simulink model "SingleHip_R2013a"  (R2013a)
settings: Solver=FixedStepDiscrete  StartTime=0.0  StopTime=inf  FixedStep=0.001  MaxStep=0.001  RelTol=1e-3
libraries: xpcethercatlib x21, dspswit3 x1
settings Model: xpc_rtwmakecfg_data=_xpcethercatlib_  BufferReuse=off  Creator=bgbuss  LastModifiedBy=bgbuss
settings OptimizationCC: BlockReduction=off  OptimizeBlockIOStorage=off  BufferReuse=off  ExpressionFolding=off  LocalBlockOutputs=off
settings DebuggingCC: UnderspecifiedInitializationDetection=Simplified
settings HardwareCC: ProdIntDivRoundTo=Zero  ProdEndianess=LittleEndian  ProdHWDeviceType=Generic->32-bit x86 compatible
settings RTWCC: SystemTargetFile=xpctarget.tlc  TemplateMakefile=xpc_default_tmf  Description=xPC Target  ProcessScript=xpctarget_make_rtw_hook  RTWCompilerOptimization=On
settings CodeAppCC: MATLABSourceComments=on
settings xpcTargetCC: TargetFcnLib=ansi_tfl_table_tmw.mat  CodeReplacementLibrary=XPC_BLAS  ParMdlRefBuildCompliant=on  ConcurrentExecutionCompliant=on  CombineSignalStateStructs=off  MATLABClassNameForMDSCustomization=xpcAperiodicCustomization  GRTInterface=on  GenerateAllocFcn=off  RL32LogBufSizeModifier=100000000  xPCTaskExecutionProfile=off  xPCRL32EventNumber=5000  xPCisModelTimeout=off  xPCModelTimeoutSecs=20  xPCLoadParamSetFile=off  xPCConcurrentTasks=off  xPCEnableSFAnimation=off

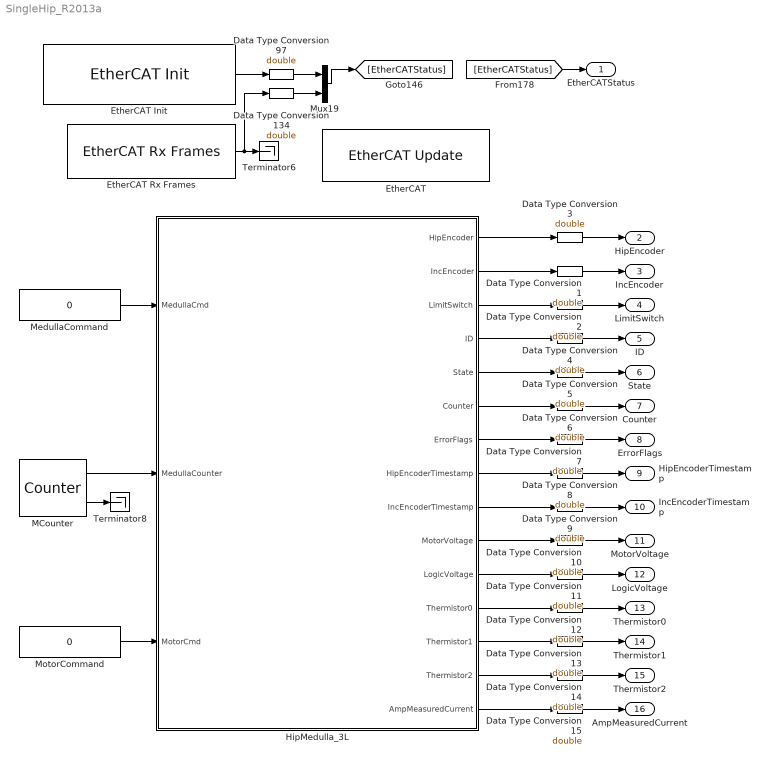
== system SingleHip_R2013a ==
  Data Type Conversion{1..15,97,134} (17 alike) : DataTypeConversion  OutDataTypeStr=double
  EtherCAT : xpcethercatlib/EtherCAT Update   Priority=4  device_id=0  task_id_list=[1]  task_rates=[1]  task_priorities=[1500]
  "EtherCAT Init " : xpcethercatlib/EtherCAT Init   Priority=0  config_file='20140605FullWithMicrostrainDC-eni.xml'  device_id=0  pci_bus=10  pci_slot=0  enaDC=on  errRptLevel=0  sample_time=-1
  EtherCAT Rx Frames : xpcethercatlib/EtherCAT Rx Frames   Priority=1  device_id=0  sample_time=0
  HipMedulla_3L : Subsystem
  MCounter : dspswit3/Counter  Direction=Up  CountEvent=Free running  CounterSize=User defined  MaxCount=65535  InitialCount=0  Output=Count and Hit  HitValue=32  ResetInput=off  SamplesPerFrame=1  Ts=.001  CntDtype=double  HitDtype=Logical
  MedullaCommand : Constant  Value=0
  MotorCommand : Constant  Value=0
  Mux19 : Mux  Inputs=2
  Terminator6 : Terminator
  Terminator8 : Terminator
  EtherCATStatus : Outport
  HipEncoder : Outport  Port=2
  IncEncoder : Outport  Port=3
  LimitSwitch : Outport  Port=4
  ID : Outport  Port=5
  State : Outport  Port=6
  Counter : Outport  Port=7
  ErrorFlags : Outport  Port=8
  HipEncoderTimestamp : Outport  Port=9
  IncEncoderTimestamp : Outport  Port=10
  MotorVoltage : Outport  Port=11
  LogicVoltage : Outport  Port=12
  Thermistor0 : Outport  Port=13
  Thermistor1 : Outport  Port=14
  Thermistor2 : Outport  Port=15
  AmpMeasuredCurrent : Outport  Port=16
  wires:
  Data Type Conversion3/1 -> HipEncoder/1
  [EtherCATStatus] -> EtherCATStatus/1
  Mux19/1 -> [EtherCATStatus]
  "EtherCAT Init "/1 -> Data Type Conversion97/1
  HipMedulla_3L/2(IncEncoder) -> Data Type Conversion1/1
  HipMedulla_3L/3(LimitSwitch) -> Data Type Conversion2/1
  HipMedulla_3L/4(ID) -> Data Type Conversion4/1
  HipMedulla_3L/5(State) -> Data Type Conversion5/1
  HipMedulla_3L/6(Counter) -> Data Type Conversion6/1
  HipMedulla_3L/7(ErrorFlags) -> Data Type Conversion7/1
  HipMedulla_3L/8(HipEncoderTimestamp) -> Data Type Conversion8/1
  HipMedulla_3L/9(IncEncoderTimestamp) -> Data Type Conversion9/1
  HipMedulla_3L/10(MotorVoltage) -> Data Type Conversion10/1
  HipMedulla_3L/11(LogicVoltage) -> Data Type Conversion11/1
  HipMedulla_3L/12(Thermistor0) -> Data Type Conversion12/1
  HipMedulla_3L/13(Thermistor1) -> Data Type Conversion13/1
  HipMedulla_3L/14(Thermistor2) -> Data Type Conversion14/1
  HipMedulla_3L/15(AmpMeasuredCurrent) -> Data Type Conversion15/1
  EtherCAT Rx Frames/1 -> Data Type Conversion134/1, Terminator6/1
  MCounter/2 -> Terminator8/1
  HipMedulla_3L/1(HipEncoder) -> Data Type Conversion3/1
  Data Type Conversion5/1 -> State/1
  Data Type Conversion6/1 -> Counter/1
  Data Type Conversion7/1 -> ErrorFlags/1
  Data Type Conversion8/1 -> HipEncoderTimestamp/1
  Data Type Conversion9/1 -> IncEncoderTimestamp/1
  Data Type Conversion10/1 -> MotorVoltage/1
  Data Type Conversion11/1 -> LogicVoltage/1
  Data Type Conversion12/1 -> Thermistor0/1
  Data Type Conversion13/1 -> Thermistor1/1
  Data Type Conversion14/1 -> Thermistor2/1
  Data Type Conversion15/1 -> AmpMeasuredCurrent/1
  MCounter/1 -> HipMedulla_3L/2(MedullaCounter)
  MedullaCommand/1 -> HipMedulla_3L/1(MedullaCmd)
  MotorCommand/1 -> HipMedulla_3L/3(MotorCmd)
  Data Type Conversion2/1 -> LimitSwitch/1
  Data Type Conversion4/1 -> ID/1
  Data Type Conversion1/1 -> IncEncoder/1
  Data Type Conversion97/1 -> Mux19/1
  Data Type Conversion134/1 -> Mux19/2

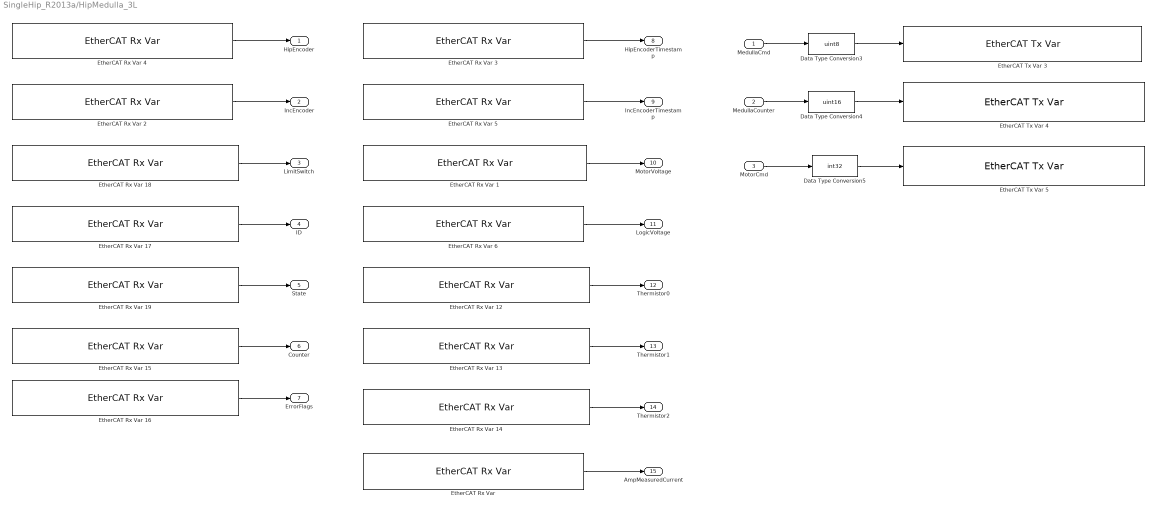
== system SingleHip_R2013a/HipMedulla_3L ==
  MedullaCmd : Inport
  MedullaCounter : Inport  Port=2
  MotorCmd : Inport  Port=3
  Data Type Conversion3 : DataTypeConversion  OutDataTypeStr=uint8
  Data Type Conversion4 : DataTypeConversion  OutDataTypeStr=uint16
  Data Type Conversion5 : DataTypeConversion  OutDataTypeStr=int32
  "EtherCAT Rx Var " : xpcethercatlib/EtherCAT Rx Var   Priority=2  sig_name=Box 6 (ATRIAS 2.1 Hip (Medulla 1.5)).Measured Current.Amp Measured Current  sig_offset=2480  sig_type=int16  type_size=16  sig_dim=1  device_id=0  sample_time=0.001000
  EtherCAT Rx Var 1 : xpcethercatlib/EtherCAT Rx Var   Priority=2  sig_name=Box 6 (ATRIAS 2.1 Hip (Medulla 1.5)).Power.Motor Voltage  sig_offset=2400  sig_type=uint16  type_size=16  sig_dim=1  device_id=0  sample_time=0.001000
  EtherCAT Rx Var 12 : xpcethercatlib/EtherCAT Rx Var   Priority=2  sig_name=Box 6 (ATRIAS 2.1 Hip (Medulla 1.5)).Thermistors.Thermistor 0  sig_offset=2432  sig_type=uint16  type_size=16  sig_dim=1  device_id=0  sample_time=0.001000
  EtherCAT Rx Var 13 : xpcethercatlib/EtherCAT Rx Var   Priority=2  sig_name=Box 6 (ATRIAS 2.1 Hip (Medulla 1.5)).Thermistors.Thermistor 1  sig_offset=2448  sig_type=uint16  type_size=16  sig_dim=1  device_id=0  sample_time=0.001000
  EtherCAT Rx Var 14 : xpcethercatlib/EtherCAT Rx Var   Priority=2  sig_name=Box 6 (ATRIAS 2.1 Hip (Medulla 1.5)).Thermistors.Thermistor 2  sig_offset=2464  sig_type=uint16  type_size=16  sig_dim=1  device_id=0  sample_time=0.001000
  EtherCAT Rx Var 15 : xpcethercatlib/EtherCAT Rx Var   Priority=2  sig_name=Box 6 (ATRIAS 2.1 Hip (Medulla 1.5)).uController Status.Counter  sig_offset=2328  sig_type=uint8  type_size=8  sig_dim=1  device_id=0  sample_time=0.001000
  EtherCAT Rx Var 16 : xpcethercatlib/EtherCAT Rx Var   Priority=2  sig_name=Box 6 (ATRIAS 2.1 Hip (Medulla 1.5)).uController Status.Error Flags  sig_offset=2336  sig_type=uint8  type_size=8  sig_dim=1  device_id=0  sample_time=0.001000
  EtherCAT Rx Var 17 : xpcethercatlib/EtherCAT Rx Var   Priority=2  sig_name=Box 6 (ATRIAS 2.1 Hip (Medulla 1.5)).uController Status.ID  sig_offset=2312  sig_type=uint8  type_size=8  sig_dim=1  device_id=0  sample_time=0.001000
  EtherCAT Rx Var 18 : xpcethercatlib/EtherCAT Rx Var   Priority=2  sig_name=Box 6 (ATRIAS 2.1 Hip (Medulla 1.5)).uController Status.Limit Switch  sig_offset=2344  sig_type=uint8  type_size=8  sig_dim=1  device_id=0  sample_time=0.001000
  EtherCAT Rx Var 19 : xpcethercatlib/EtherCAT Rx Var   Priority=2  sig_name=Box 6 (ATRIAS 2.1 Hip (Medulla 1.5)).uController Status.State  sig_offset=2320  sig_type=uint8  type_size=8  sig_dim=1  device_id=0  sample_time=0.001000
  EtherCAT Rx Var 2 : xpcethercatlib/EtherCAT Rx Var   Priority=2  sig_name=Box 6 (ATRIAS 2.1 Hip (Medulla 1.5)).Incremental Encoder.Incremental Encoder  sig_offset=2496  sig_type=uint16  type_size=16  sig_dim=1  device_id=0  sample_time=0.001000
  EtherCAT Rx Var 3 : xpcethercatlib/EtherCAT Rx Var   Priority=2  sig_name=Box 6 (ATRIAS 2.1 Hip (Medulla 1.5)).Hip Encoder.Timestamp  sig_offset=2384  sig_type=uint16  type_size=16  sig_dim=1  device_id=0  sample_time=0.001000
  EtherCAT Rx Var 4 : xpcethercatlib/EtherCAT Rx Var   Priority=2  sig_name=Box 6 (ATRIAS 2.1 Hip (Medulla 1.5)).Hip Encoder.Encoder  sig_offset=2352  sig_type=uint32  type_size=32  sig_dim=1  device_id=0  sample_time=0.001000
  EtherCAT Rx Var 5 : xpcethercatlib/EtherCAT Rx Var   Priority=2  sig_name=Box 6 (ATRIAS 2.1 Hip (Medulla 1.5)).Incremental Encoder.Incremental Encoder Timestamp  sig_offset=2512  sig_type=uint16  type_size=16  sig_dim=1  device_id=0  sample_time=0.001000
  EtherCAT Rx Var 6 : xpcethercatlib/EtherCAT Rx Var   Priority=2  sig_name=Box 6 (ATRIAS 2.1 Hip (Medulla 1.5)).Power.Logic Voltage  sig_offset=2416  sig_type=uint16  type_size=16  sig_dim=1  device_id=0  sample_time=0.001000
  EtherCAT Tx Var 3 : xpcethercatlib/EtherCAT Tx Var   Priority=3  sig_name=Box 6 (ATRIAS 2.1 Hip (Medulla 1.5)).uControllerInput.Command  sig_offset=2312  sig_type=uint8  type_size=8  sig_dim=1  device_id=0  sample_time=0.001000
  EtherCAT Tx Var 4 : xpcethercatlib/EtherCAT Tx Var   Priority=3  sig_name=Box 6 (ATRIAS 2.1 Hip (Medulla 1.5)).uControllerInput.Counter  sig_offset=2320  sig_type=uint16  type_size=16  sig_dim=1  device_id=0  sample_time=0.001000
  EtherCAT Tx Var 5 : xpcethercatlib/EtherCAT Tx Var   Priority=3  sig_name=Box 6 (ATRIAS 2.1 Hip (Medulla 1.5)).uControllerInput.Motor Current  sig_offset=2336  sig_type=int32  type_size=32  sig_dim=1  device_id=0  sample_time=0.001000
  HipEncoder : Outport
  IncEncoder : Outport  Port=2
  LimitSwitch : Outport  Port=3
  ID : Outport  Port=4
  State : Outport  Port=5
  Counter : Outport  Port=6
  ErrorFlags : Outport  Port=7
  HipEncoderTimestamp : Outport  Port=8
  IncEncoderTimestamp : Outport  Port=9
  MotorVoltage : Outport  Port=10
  LogicVoltage : Outport  Port=11
  Thermistor0 : Outport  Port=12
  Thermistor1 : Outport  Port=13
  Thermistor2 : Outport  Port=14
  AmpMeasuredCurrent : Outport  Port=15
  wires:
  Data Type Conversion3/1 -> EtherCAT Tx Var 3/1
  Data Type Conversion4/1 -> EtherCAT Tx Var 4/1
  Data Type Conversion5/1 -> EtherCAT Tx Var 5/1
  MedullaCmd/1 -> Data Type Conversion3/1
  MedullaCounter/1 -> Data Type Conversion4/1
  MotorCmd/1 -> Data Type Conversion5/1
  EtherCAT Rx Var 5/1 -> IncEncoderTimestamp/1
  EtherCAT Rx Var 4/1 -> HipEncoder/1
  EtherCAT Rx Var 3/1 -> HipEncoderTimestamp/1
  EtherCAT Rx Var 2/1 -> IncEncoder/1
  EtherCAT Rx Var 15/1 -> Counter/1
  EtherCAT Rx Var 17/1 -> ID/1
  EtherCAT Rx Var 18/1 -> LimitSwitch/1
  EtherCAT Rx Var 19/1 -> State/1
  EtherCAT Rx Var 16/1 -> ErrorFlags/1
  EtherCAT Rx Var 6/1 -> LogicVoltage/1
  EtherCAT Rx Var 1/1 -> MotorVoltage/1
  EtherCAT Rx Var 12/1 -> Thermistor0/1
  EtherCAT Rx Var 13/1 -> Thermistor1/1
  EtherCAT Rx Var 14/1 -> Thermistor2/1
  "EtherCAT Rx Var "/1 -> AmpMeasuredCurrent/1
